simulink model "Hunter_gazebo_call"  (R2023a)
settings: Solver=ode3  StartTime=0.0  StopTime=inf  FixedStep=0.05  RelTol=1e-3  EnableMultiTasking=on
InitFcn:
  | rosshutdown
  | rosinit("http://localhost:11311")
model workspace (MAT data in the model file):
  SL_ROS_VariableLengthArrays_MaxSizes : object (value not decoded)
values from neighbouring files (symbols this model uses):
  roi = [0, 7, -7, 7, -1, 2]    [TrackExample_sim.m]
undefined symbols (not defined in the file or in its folder): Angular, L, Ld, Linear
libraries: robotlib x20, slpidlib x4, robotalgslib x3, slctrlblks x2, mobileRoboticsLib x2, robotcorelib x2, simulink_extras x2
(part 2 of 2)

== matlab function Hunter_gazebo_call/old version/Generate New Path /Generate New Waypoint/extractConeBboxs_l ==
  data: y_coneBboxs_l output size=[50 4]; bboxData input; len input; b_coneBboxs_l output size=[50 4]
function [y_coneBboxs_l, b_coneBboxs_l] = extractConesBboxs_l(bboxData, len)

    temp_y_coneBboxs = zeros(len,4);
    temp_b_coneBboxs = zeros(len,4);

    y_count = 0;
    b_count = 0;

    % disp(len)
    for i = 1:len
        x = bboxData.ObjectList.Detections(i).Mask.Roi.X;
        y = bboxData.ObjectList.Detections(i).Mask.Roi.Y;
        w = bboxData.ObjectList.Detections(i).Mask.Roi.Width;
        h = bboxData.ObjectList.Detections(i).Mask.Roi.Height;

        label = char(bboxData.ObjectList.Detections(i).Label)';
        label = label(:,1:6);
        
        if strcmp(label,'y_cone')
            y_count = y_count + 1;
            temp_y_coneBboxs(y_count,:) = [x y w h];
        elseif strcmp(label,'b_cone')
            b_count = b_count + 1;
            temp_b_coneBboxs(b_count,:) = [x y w h];
        else
            disp("No");
        end
    end
   
    y_coneBboxs_l = temp_y_coneBboxs(1:y_count, :);
    b_coneBboxs_l = temp_b_coneBboxs(1:b_count, :);
   
end

== matlab function Hunter_gazebo_call/old version/Generate New Path /Generate New Waypoint/generate_waypoints ==
  data: PtCloudData input single size=[3000 3]; y_coneBboxs_l input; b_coneBboxs_l input; y_coneBboxs_r input; b_coneBboxs_r input; wp_x output size=[50,1]; wp_y output size=[50,1]
function [wp_x, wp_y] = generate_waypoints(PtCloudData, y_coneBboxs_l, b_coneBboxs_l,y_coneBboxs_r, b_coneBboxs_r)
    

    % tic
    %#codegen
    coder.extrinsic("FinalFulltrack");
    wp_x = double(zeros(50,1));
    wp_y = double(zeros(50,1));

    [wp_x, wp_y] = FinalFulltrack(PtCloudData, y_coneBboxs_l, b_coneBboxs_l, y_coneBboxs_r, b_coneBboxs_r);
    % disp(toc)
   
end

== matlab function Hunter_gazebo_call/old version/MATLAB Function3 ==
  data: waypoints input; u2 output; currentPose input
function u2 = checkDist(waypoints, currentPose)

   if norm(waypoints(end,:) - [currentPose(1) currentPose(2)]) < 2
       u2 = 0;  % generate new waypoints
   else
       u2 = 1;  % follow existing waypoints
   end

== matlab function Hunter_gazebo_call/old version/MATLAB Function4 ==
  data: odomWP input; u1 output
function u1 = checkWP(odomWP)
    
        
    if isempty(find(odomWP))
        u1 = 0;  % generate new waypoint
    else
        u1 = 1;  % follow existing waypoint
    end

end

== matlab function Hunter_gazebo_call/Generate New Path /Generate New Waypoint/extractConesBboxs_r ==
  data: y_coneBboxs_r output size=[50 4]; bboxData input; len input; b_coneBboxs_r output size=[50 4]
function [y_coneBboxs_r,b_coneBboxs_r] = extractConesBboxs_r(bboxData, len)

    temp_y_coneBboxs = zeros(len,4);
    temp_b_coneBboxs = zeros(len,4);

    y_count = 0;
    b_count = 0;

    % disp(len)
    for i = 1:len
        x = bboxData.ObjectList.Detections(i).Mask.Roi.X;
        y = bboxData.ObjectList.Detections(i).Mask.Roi.Y;
        w = bboxData.ObjectList.Detections(i).Mask.Roi.Width;
        h = bboxData.ObjectList.Detections(i).Mask.Roi.Height;

        label = char(bboxData.ObjectList.Detections(i).Label)';
        label = label(:,1:6);
        
        if strcmp(label,'y_cone')
            y_count = y_count + 1;
            temp_y_coneBboxs(y_count,:) = [x y w h];
        elseif strcmp(label,'b_cone')
            b_count = b_count + 1;
            temp_b_coneBboxs(b_count,:) = [x y w h];
        else
            disp("No");
        end
    end
   
    y_coneBboxs_r = temp_y_coneBboxs(1:y_count, :);
    b_coneBboxs_r = temp_b_coneBboxs(1:b_count, :);
   
end
